simulink model "OpenLoopModel"  (R2019b)
settings: Solver=FixedStepAuto  StartTime=0.0  StopTime=10.0  FixedStep=0.01  RelTol=1e-3
undefined symbols (not defined in the file or in its folder): A_real, B_real, C_real, sigbuilder_block, x_0
settings Model: Creator=miche  LastModifiedBy=miche

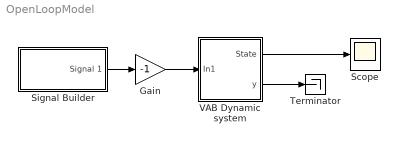
== system OpenLoopModel ==
  Gain : Gain  Gain=-1
  Scope : Scope
  Signal Builder : Subsystem  Tag=STV Subsys  LoadFcn=sigbuilder_block('load');  StartFcn=sigbuilder_block('start');  StopFcn=sigbuilder_block('stop');  ClipboardFcn=sigbuilder_block('clipboard');  mask(Sigbuilder block){tuvar=[0:10]}
      mask help: Simulink:masks:SigbuilderBlock_MD
      mask init:
      | if ~strcmp(get_param(bdroot(gcbh),'SimulationStatus'),'stopped') tuvar = sigbuilder_block('maskInit'); end
      settings: CopyFcn=sigbuilder_block('copy');  DeleteFcn=sigbuilder_block('delete');  ModelCloseFcn=sigbuilder_block('modelClose');  PreSaveFcn=sigbuilder_block('preSave');  PauseFcn=sigbuilder_block('pause');  ContinueFcn=sigbuilder_block('continue');  NameChangeFcn=sigbuilder_block('namechange');  OpenFcn=sigbuilder_block('open',[1024.5 -211.5 1440 729.75 ]);  CloseFcn=sigbuilder_block('close');
      mask Display: plot(0, 0, 100, 100,[2, 2, 32, 32, 2], [68, 8, 8, 68, 68],[32, 2], [38, 38], [32, 19, 2],[53, 60, 44], [32, 17, 17, 2],[16, 16, 31, 31]);txt = getActiveGroup(gcbh);text(2, 100, txt,'verticalAlignment', 'top');
  Terminator : Terminator
  VAB Dynamic system : Subsystem
  wires:
  VAB Dynamic system/2(y) -> Terminator/1
  VAB Dynamic system/1(State) -> Scope/1
  Signal Builder/1(Signal 1) -> Gain/1
  Gain/1 -> VAB Dynamic system/1(In1)

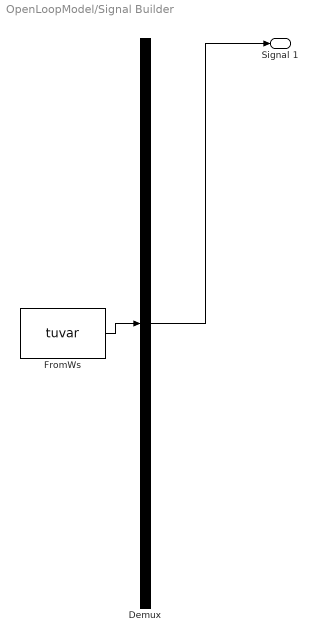
== system OpenLoopModel/Signal Builder ==
  Demux : Demux  Tag=STV Demux  Outputs=1
  FromWs : FromWorkspace  Tag=STV FromWs  VariableName=tuvar  SampleTime=0
      SigBuilderData=|
      | common.afterFinalStr = 'Extrapolate'
      | common.sampleTime = 0
      | dataSet.timeRange = [0 10]
      | dataSet.name = 'Group 1'
      | sbobj.Groups.Name = 'Group 1'
      | sbobj.Groups.Signals.Name = 'Signal 1'
      | sbobj.Groups.Signals.XData = [0 4 4 4.58 4.58 10]
      | sbobj.Groups.Signals.YData = [0 0 0.998 1 0 0]
  Signal 1 : Outport  Tag=STV Outport
  wires:
  Demux/1 -> Signal 1/1
  FromWs/1 -> Demux/1

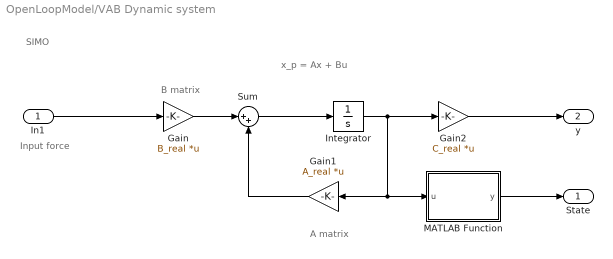
== system OpenLoopModel/VAB Dynamic system ==
  note: SIMO
  note: x_p = Ax + Bu
  note: B matrix
  note: A matrix
  note: Input force
  In1 : Inport
  Gain : Gain  Gain=B_real  Multiplication=Matrix(K*u)
  Gain1 : Gain  Gain=A_real  Multiplication=Matrix(K*u)
  Gain2 : Gain  Gain=C_real  Multiplication=Matrix(K*u) (u vector)
  Integrator : Integrator  InitialCondition=x_0
  MATLAB Function : MATLAB Function  TreatAsAtomicUnit=on
  Sum : Sum  Inputs=|++
  State : Outport
  y : Outport  Port=2
  wires:
  Gain2/1 -> y/1
  Gain1/1 -> Sum/2
  Integrator/1 -> Gain2/1, MATLAB Function/1(u), Gain1/1
  Gain/1 -> Sum/1
  In1/1 -> Gain/1
  Sum/1 -> Integrator/1
  MATLAB Function/1(y) -> State/1

== matlab function OpenLoopModel/VAB Dynamic system/MATLAB Function ==
  data: u input; y output
function y = fcn(u)

if u(3) ~= 0
   u(3) = mod(u(3), 2 * pi); 
end

y = rad2deg(u(3));
